simulink model "dPTPUDPNode1_tm"  (R2018b)
settings: Solver=FixedStepDiscrete  StartTime=0.0  StopTime=inf  FixedStep=0.01  RelTol=1e-3  EnableMultiTasking=on
undefined symbols (not defined in the file): ipaddr, PTP
libraries: xpcutilitieslib x6, xpcrtudplib x6, ptplib x5, slrtlib x4
settings Model: SimulationMode=external  Creator=The MathWorks, Inc.  LastModifiedBy=MAE-NCSUCORE
settings SolverCC: ConcurrentTasks=on  AutoInsertRateTranBlk=on  DecoupledContinuousIntegration=on  MinimalZcImpactIntegration=on
settings DataIOCC: SaveFormat=StructureWithTime
settings OptimizationCC: BlockReduction=off  OptimizeBlockIOStorage=off  BufferReuse=off  GlobalBufferReuse=off  ExpressionFolding=off  LocalBlockOutputs=off  OptimizeDataStoreBuffers=off  BusAssignmentInplaceUpdate=off
settings DebuggingCC: LibraryContextMissingDiagnostic=none
settings HardwareCC: ProdBitPerPointer=32  ProdBitPerSizeT=32  ProdBitPerPtrDiffT=32  ProdLargestAtomicFloat=None  ProdWordSize=32  ProdLongLongMode=on  ProdHWDeviceType=Generic->32-bit x86 compatible
settings SFSimCC: SimUseLocalCustomCode=off
settings RTWCC: SystemTargetFile=slrt.tlc  TemplateMakefile=slrt_default_tmf  Description=Simulink Real-Time  RTWVerbose=off  RTWUseLocalCustomCode=off  CodeExecutionProfiling=on  RTWCompilerOptimization=on
settings SimulinkRealTimeCC: SupportVariableSizeSignals=on  PreserveStateflowLocalDataDimensions=off  RL32LogTETModifier=off  RL32ObjectName=tg1  xPCisDefaultEnv=off  xPCTargetPCEnvName=Machine2  xPCConcurrentTasks=on

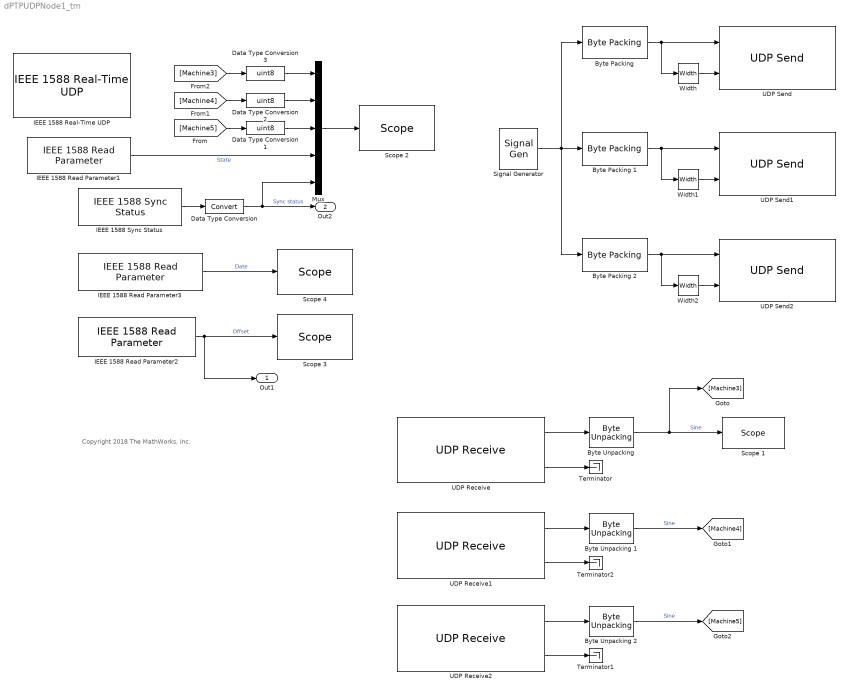
== system dPTPUDPNode1_tm ==
  note: Copyright 2018 The MathWorks, Inc.
  "Byte Packing " : xpcutilitieslib/Byte Packing   MaskPackedDataType=uint8  MaskUnpackedDataTypes={'double'}  MaskAlignment=1
  Byte Packing 1 : xpcutilitieslib/Byte Packing   MaskPackedDataType=uint8  MaskUnpackedDataTypes={'double'}  MaskAlignment=1
  Byte Packing 2 : xpcutilitieslib/Byte Packing   MaskPackedDataType=uint8  MaskUnpackedDataTypes={'double'}  MaskAlignment=1
  "Byte Unpacking " : xpcutilitieslib/Byte Unpacking   MaskUnpackedDataTypes={'double'}  MaskUnpackedDataSizes={[1]}  MaskAlignment=1
      settings: SourceProductName=Simulink Real-Time  SourceProductBaseCode=XP
  Byte Unpacking 1 : xpcutilitieslib/Byte Unpacking   MaskUnpackedDataTypes={'double'}  MaskUnpackedDataSizes={[1]}  MaskAlignment=1
      settings: SourceProductName=Simulink Real-Time  SourceProductBaseCode=XP
  Byte Unpacking 2 : xpcutilitieslib/Byte Unpacking   MaskUnpackedDataTypes={'double'}  MaskUnpackedDataSizes={[1]}  MaskAlignment=1
      settings: SourceProductName=Simulink Real-Time  SourceProductBaseCode=XP
  Data Type Conversion : DataTypeConversion
  Data Type Conversion1 : DataTypeConversion  OutDataTypeStr=uint8
  Data Type Conversion2 : DataTypeConversion  OutDataTypeStr=uint8
  Data Type Conversion3 : DataTypeConversion  OutDataTypeStr=uint8
  IEEE 1588 Read Parameter1 : ptplib/IEEE 1588 Read Parameter  Priority=1  ID=1  param=Protocol state  sample_time=0.01  enable_read_precision=off
      settings: SourceProductName=Simulink Real-Time  SourceProductBaseCode=XP
  IEEE 1588 Read Parameter2 : ptplib/IEEE 1588 Read Parameter  Priority=1  ID=1  param=Offset from Master  sample_time=0.01  enable_read_precision=off
      settings: SourceProductName=Simulink Real-Time  SourceProductBaseCode=XP
  IEEE 1588 Read Parameter3 : ptplib/IEEE 1588 Read Parameter  Priority=1  ID=1  param=PTP time (time-of-day)  sample_time=0.01  enable_read_precision=off
      settings: SourceProductName=Simulink Real-Time  SourceProductBaseCode=XP
  IEEE 1588 Sync Status : ptplib/IEEE 1588 Sync Status  Priority=1  ID=1  offset_threshold=250e-6  sample_time=0.01
      settings: SourceProductName=Simulink Real-Time  SourceProductBaseCode=XP
  IEEE 1588 Real-Time UDP : ptplib/IEEE 1588 Real-Time UDP  Priority=0  ID=1  PciBus=2  PciSlot=0  PciFunction=0  time_inc=4000000  sample_time=0.01  IpSource=Specify  IpAddress=30.30.30.30  SubnetMask=255.255.255.0  Gateway=0.0.0.0  Receive1=0.0.0.0  dest_ip_select=Specify  custom_dest_ip_addr=255.255.255.255  MulticastList=[ipaddr('224.0.1.129'), ipaddr('224.0.0.107')]  Multicast={macaddr('01:00:5E:00:01:81'), macaddr('01:00:5E:00:00:6B')}  time_source=Ethernet board  timescale=PTP (1970-01-01)  epoch=[1970 01 01 00]  delay_measure=Request-response  slave_only=off  enable_advanced_config=on  domain_num=0  utc_offset=35  priority1=1  clock_class=248  clock_accuracy=hex2dec('FE')  priority2=1  announce_interval=1  sync_interval=0.05  min_pdelay_req_interval=0.1  announce_receipt_timeout=3
      settings: SourceProductName=Simulink Real-Time  SourceProductBaseCode=XP
  Mux : Mux  Inputs=5
  Scope 1 : slrtlib/Displays and Logging/Scope   scopeno=4  scopetype=Target  autostart=on  viewmode=Graphical rolling  formatstr='%15.6f'  grid=on  ylimits=[0,0]  nosamples=250  noprepostsamples=0  interleave=1  triggermode=FreeRun  triggersignal=1  trigsignalfromport=off  triggerlevel=0.0  triggerslope=Either  triggerscope=1  triggersample=0  filename=data.dat  mode=Lazy  writesize=512  autorestart=off  dynamicfilemode=off  maxwritefilesize=512*1024^2
  Scope 2 : slrtlib/Displays and Logging/Scope   scopeno=1  scopetype=Target  autostart=on  viewmode=Numerical  formatstr='%15.6f'  grid=on  ylimits=[0,0]  nosamples=3  noprepostsamples=0  interleave=1  triggermode=FreeRun  triggersignal=1  trigsignalfromport=off  triggerlevel=0.0  triggerslope=Either  triggerscope=1  triggersample=0  filename=data.dat  mode=Lazy  writesize=512  autorestart=off  dynamicfilemode=off  maxwritefilesize=512*1024^2
  Scope 3 : slrtlib/Displays and Logging/Scope   scopeno=3  scopetype=Target  autostart=on  viewmode=Graphical rolling  formatstr='%15.6f'  grid=on  ylimits=[0,0]  nosamples=250  noprepostsamples=0  interleave=1  triggermode=FreeRun  triggersignal=1  trigsignalfromport=off  triggerlevel=0.0  triggerslope=Either  triggerscope=1  triggersample=0  filename=data.dat  mode=Lazy  writesize=512  autorestart=off  dynamicfilemode=off  maxwritefilesize=512*1024^2
  Scope 4 : slrtlib/Displays and Logging/Scope   scopeno=2  scopetype=Target  autostart=on  viewmode=Numerical  formatstr="'Year:            %-4.0f, Month:           %-4.0f, Day of week:     %-4.0f, Day:             %-4.0f, Hour:            %-4.0f, Minute:          %-4.0f, Second:          %-4.0f, Millisecond:     %-4.0f'"  grid=on  ylimits=[0,0]  nosamples=3  noprepostsamples=0  interleave=1  triggermode=FreeRun  triggersignal=1  trigsignalfromport=off  triggerlevel=0.0  triggerslope=Either  triggerscope=1  triggersample=0  filename=data.dat  mode=Lazy  writesize=512  autorestart=off  dynamicfilemode=off  maxwritefilesize=512*1024^2
  Signal Generator : SignalGenerator  WaveForm=square  Amplitude=10  Frequency=10  Units=rad/sec
  Terminator : Terminator
  Terminator1 : Terminator
  Terminator2 : Terminator
  UDP Receive : xpcrtudplib/UDP Receive  ipAddressVal=30.30.30.30  localPort=8001  rcvWidth=8  rcvFmAny=off  fmAddress=30.30.30.1  rcvMulticast=off  multicastAddress={30.30.30.1, 30.30.30.2, 30.30.30.3}  maxUDPQueue=8  sampleTime=0.01
      settings: SourceProductName=Simulink Real-Time
  UDP Receive1 : xpcrtudplib/UDP Receive  ipAddressVal=30.30.30.30  localPort=8002  rcvWidth=8  rcvFmAny=off  fmAddress=30.30.30.2  rcvMulticast=off  multicastAddress={30.30.30.1, 30.30.30.2, 30.30.30.3}  maxUDPQueue=8  sampleTime=0.01
      settings: SourceProductName=Simulink Real-Time
  UDP Receive2 : xpcrtudplib/UDP Receive  ipAddressVal=30.30.30.30  localPort=8003  rcvWidth=8  rcvFmAny=off  fmAddress=30.30.30.3  rcvMulticast=off  multicastAddress={30.30.30.1, 30.30.30.2, 30.30.30.3}  maxUDPQueue=8  sampleTime=0.01
      settings: SourceProductName=Simulink Real-Time
  UDP Send : xpcrtudplib/UDP Send  ipAddressVal=30.30.30.30  localPort=8001  toAddress=30.30.30.1  toPort=8000  sampleTime=0.01
      settings: SourceProductName=Simulink Real-Time  SourceProductBaseCode=XP
  UDP Send1 : xpcrtudplib/UDP Send  ipAddressVal=30.30.30.30  localPort=8002  toAddress=30.30.30.2  toPort=8000  sampleTime=0.01
      settings: SourceProductName=Simulink Real-Time  SourceProductBaseCode=XP
  UDP Send2 : xpcrtudplib/UDP Send  ipAddressVal=30.30.30.30  localPort=8003  toAddress=30.30.30.3  toPort=8000  sampleTime=0.01
      settings: SourceProductName=Simulink Real-Time  SourceProductBaseCode=XP
  Width : Width
  Width1 : Width
  Width2 : Width
  Out1 : Outport
  Out2 : Outport  Port=2
  wires:
  IEEE 1588 Read Parameter3/1 -> Scope 4/1  "Date"
  "Byte Packing "/1 -> Width/1, UDP Send/1
  Width/1 -> UDP Send/2
  UDP Receive/1 -> "Byte Unpacking "/1
  UDP Receive/2 -> Terminator/1
  "Byte Unpacking "/1 -> [Machine3], Scope 1/1  "Sine"
  IEEE 1588 Read Parameter2/1 -> Out1/1, Scope 3/1  "Offset"
  Mux/1 -> Scope 2/1
  IEEE 1588 Sync Status/1 -> Data Type Conversion/1
  Data Type Conversion/1 -> Mux/5, Out2/1  "Sync status"
  UDP Receive1/2 -> Terminator2/1
  UDP Receive2/2 -> Terminator1/1
  UDP Receive2/1 -> Byte Unpacking 2/1
  UDP Receive1/1 -> Byte Unpacking 1/1
  IEEE 1588 Read Parameter1/1 -> Mux/4  "State"
  [Machine3] -> Data Type Conversion3/1
  [Machine4] -> Data Type Conversion2/1
  Byte Unpacking 1/1 -> [Machine4]  "Sine"
  Byte Unpacking 2/1 -> [Machine5]  "Sine"
  [Machine5] -> Data Type Conversion1/1
  Data Type Conversion1/1 -> Mux/3
  Data Type Conversion2/1 -> Mux/2
  Data Type Conversion3/1 -> Mux/1
  Byte Packing 1/1 -> Width1/1, UDP Send1/1
  Width1/1 -> UDP Send1/2
  Signal Generator/1 -> Byte Packing 2/1, "Byte Packing "/1, Byte Packing 1/1
  Byte Packing 2/1 -> Width2/1, UDP Send2/1
  Width2/1 -> UDP Send2/2
